simulink model "RBFNN"  (Simulink 10.0)
settings: Solver=VariableStepAuto  StartTime=0.0  StopTime=5  MaxStep=5e-4  RelTol=1e-3
undefined symbols (not defined in the file): ln
libraries: powerlib x14, powerlib_meascontrol x1
settings Model: Creator=guanc  LastModifiedBy=Administrator
settings SolverCC: AlgebraicLoopSolver=LineSearch
settings DataIOCC: SaveFormat=Dataset
settings OptimizationCC: LifeSpan=auto
settings DebuggingCC: UnderspecifiedInitializationDetection=Simplified  MergeDetectMultiDrivingBlocksExec=error  SFUnexpectedBacktrackingDiag=error  SFNoUnconditionalDefaultTransitionDiag=error  SFExecutionAtInitializationDiag=warning
settings HardwareCC: ProdBitPerPointer=64  ProdBitPerSizeT=64  ProdBitPerPtrDiffT=64  ProdLargestAtomicFloat=Float  ProdIntDivRoundTo=Zero  ProdEndianess=LittleEndian  ProdWordSize=64  ProdHWDeviceType=Intel->x86-64 (Windows64)
settings ModelReferenceCC: PropagateSignalLabelsOutOfModel=on
settings GRTTargetCC: TargetLangStandard=C99 (ISO)  CombineOutputUpdateFcns=on  GRTInterface=off
settings ConfigComp: CovMetricSettings=dwe  CovHtmlReporting=off  CovSaveCumulativeToWorkspaceVar=off  CovSaveSingleToWorkspaceVar=off
settings SimscapeCC: SimscapeNormalizeSystem=off

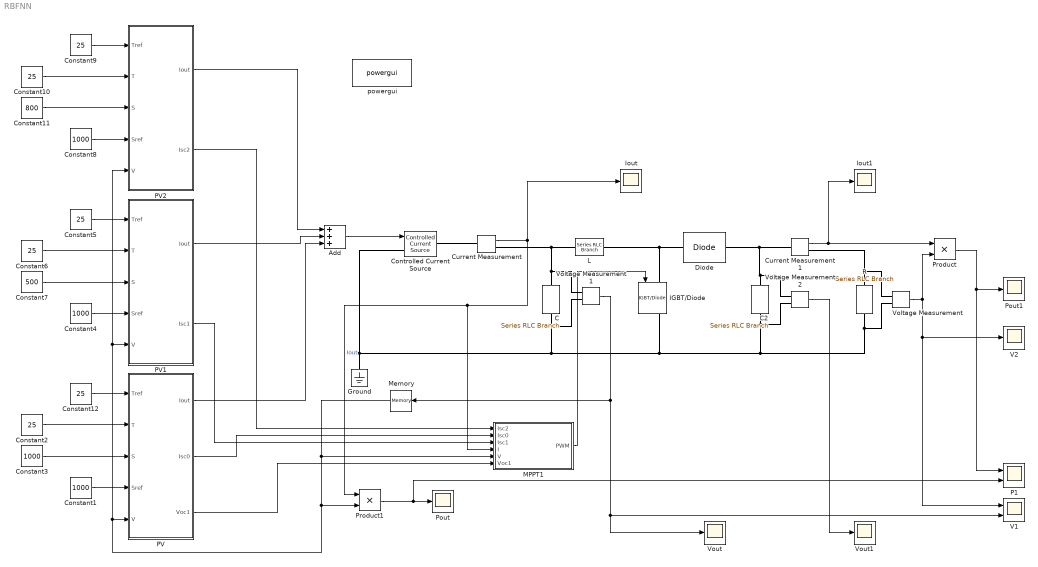
== system RBFNN ==
  Add : Sum  Inputs=+++
  C : powerlib/Elements/Series RLC Branch  LConnTagsString=__new0  RConnTagsString=__new0  BranchType=C  Resistance=1  Inductance=1e-3  SetiL0=off  InitialCurrent=0  Capacitance=47e-6  Setx0=off  InitialVoltage=1  Measurements=None
      settings: SourceProductName=Simscape Electrical
  C2 : powerlib/Elements/Series RLC Branch  LConnTagsString=__new0  RConnTagsString=__new0  BranchType=C  Resistance=1  Inductance=1e-3  SetiL0=off  InitialCurrent=0  Capacitance=470e-6  Setx0=off  InitialVoltage=1  Measurements=None
      settings: SourceProductName=Simscape Electrical
  Constant{1,3..4,8} (4 alike) : Constant  Value=1000
  Constant{2,5..6,9..10,12} (6 alike) : Constant  Value=25
  Constant11 : Constant  Value=800
  Constant7 : Constant  Value=500
  Controlled Current Source : powerlib/Electrical Sources/Controlled Current Source  Initialize=on  Source_Type=DC  Amplitude=0  Phase=0  Frequency=0  Measurements=None
      settings: SourceProductName=Simscape Electrical
  Current Measurement : powerlib/Measurements/Current Measurement  PhasorSimulation=off  OutputType=Complex  PSBequivalent=0
      settings: SourceProductName=Simscape Electrical
  Current Measurement1 : powerlib/Measurements/Current Measurement  PhasorSimulation=off  OutputType=Complex  PSBequivalent=0
      settings: SourceProductName=Simscape Electrical
  Diode : powerlib/Power Electronics/Diode  Ron=0.001  Lon=0  Vf=0.8  IC=0  UseSnubber=off  Rs=500  Cs=250e-9  Measurements=off
      settings: SourceProductName=Simscape Electrical
  Ground : powerlib/Elements/Ground  LConnTagsString=a
      settings: SourceProductName=Simscape Electrical
  IGBT/Diode : powerlib/Power Electronics/IGBT//Diode  Ron=1e-3  Rs=1e5  Cs=inf  Measurements=on
      settings: SourceProductName=Simscape Electrical
  Iout : Scope
  Iout1 : Scope
  L : powerlib/Elements/Series RLC Branch  LConnTagsString=__new0  RConnTagsString=__new0  BranchType=L  Resistance=1  Inductance=1e-3  SetiL0=off  InitialCurrent=0  Capacitance=1e-6  Setx0=off  InitialVoltage=0  Measurements=None
      settings: SourceProductName=Simscape Electrical
  MPPT1 : Subsystem
  Memory : Memory
  P1 : Scope  NumInputPorts=2
  PV : Subsystem  mask{a=0.0025, b=0.5, c=0.0028, Voc=21.8, Vm=17.7, Isc=3.64, Im=3.24}
      mask help: 根据电池铭牌参数设置
      mask TypeOptions a: a/Gain
      mask TypeOptions b: b/Gain
      mask TypeOptions c: c/Gain
      mask TypeOptions Voc: Voc/Value
      mask TypeOptions Vm: Vm/Value
      mask TypeOptions Isc: Isc/Value
      mask TypeOptions Im: Im/Value
  PV1 : Subsystem  mask{a=0.0025, b=0.5, c=0.0028, Voc=21.8, Vm=17.7, Isc=3.64, Im=3.24}
      mask help: 根据电池铭牌参数设置
      mask TypeOptions a: a/Gain
      mask TypeOptions b: b/Gain
      mask TypeOptions c: c/Gain
      mask TypeOptions Voc: Voc/Value
      mask TypeOptions Vm: Vm/Value
      mask TypeOptions Isc: Isc/Value
      mask TypeOptions Im: Im/Value
  PV2 : Subsystem  mask{a=0.0025, b=0.5, c=0.0028, Voc=21.8, Vm=17.7, Isc=3.64, Im=3.24}
      mask help: 根据电池铭牌参数设置
      mask TypeOptions a: a/Gain
      mask TypeOptions b: b/Gain
      mask TypeOptions c: c/Gain
      mask TypeOptions Voc: Voc/Value
      mask TypeOptions Vm: Vm/Value
      mask TypeOptions Isc: Isc/Value
      mask TypeOptions Im: Im/Value
  Pout : Scope
  Pout1 : Scope
  Product : Product
  Product1 : Product
  R : powerlib/Elements/Series RLC Branch  LConnTagsString=__new0  RConnTagsString=__new0  BranchType=R  Resistance=20  Inductance=1e-3  SetiL0=off  InitialCurrent=0  Capacitance=1e-6  Setx0=off  InitialVoltage=0  Measurements=None
      settings: SourceProductName=Simscape Electrical
  V1 : Scope  NumInputPorts=2
  V2 : Scope
  Voltage Measurement : powerlib/Measurements/Voltage Measurement  PhasorSimulation=off  OutputType=Complex  PSBequivalent=0
      settings: SourceProductName=Simscape Electrical
  Voltage Measurement1 : powerlib/Measurements/Voltage Measurement  PhasorSimulation=off  OutputType=Complex  PSBequivalent=0
      settings: SourceProductName=Simscape Electrical
  Voltage Measurement2 : powerlib/Measurements/Voltage Measurement  PhasorSimulation=off  OutputType=Complex  PSBequivalent=0
      settings: SourceProductName=Simscape Electrical
  Vout : Scope
  Vout1 : Scope
  powergui : powerlib/powergui  Priority=1  SimulationMode=Discrete  SampleTime=5e-6  frequency=60  Iterations=50  frequencyindice=0  Pbase=100e6  ErrMax=1e-4  UnitsV=kV  UnitsW=MW  buscounter=0  FunctionMessages=off  echomessages=off  EnableUseOfTLC=off  CurrentSourceSwitches=on  DisableSnubberDevices=off  DisableRonSwitches=off  DisableVfSwitches=off  DisplayEquations=off  AutomaticDiscreteSolvers=off  SolverType=Tustin/Backward Euler (TBE)  Interpol=off  ExternalGateDelay=off  methode=off  Ts=0  x0status=blocks  SPID=off  SwTol=0  HookPort=off  NonlinearTolerance=1e-4  nMaxIteration=100  ContinueOnMaxIteration=off  RestoreLinks=warning  ResistiveCurrentMeasurement=off  Frange=[0:2:500]  Ylog=off  Xlog=on  ShowGrid=off  save=off  variable=ZData  structure=0  ZoomFFT=off  StartTime=0.0  cycles=1  DisplayStyle=1  fundamental=60  FreqAxis=off  MaxFrequency=1000  frequencyindicesteady=1  RmsSteady=1  display=off
      settings: SourceProductName=Simscape Electrical
  wires:
  Current Measurement1/1 -> Iout1/1, Product/1
  Voltage Measurement/1 -> V2/1, V1/1, Product/2
  Product/1 -> P1/1, Pout1/1
  Current Measurement/1 -> MPPT1/4(I), Product1/1, Iout/1  "Iout"
  MPPT1/1(PWM) -> IGBT/Diode/1
  Product1/1 -> P1/2, Pout/1
  Voltage Measurement2/1 -> Vout1/1
  Voltage Measurement1/1 -> Memory/1, Vout/1, V1/2
  Constant3/1 -> PV/3(S)
  Constant12/1 -> PV/1(Tref)
  PV/1(Iout) -> Add/3
  Constant2/1 -> PV/2(T)
  Constant1/1 -> PV/4(Sref)
  Constant4/1 -> PV1/4(Sref)
  Constant6/1 -> PV1/2(T)
  Constant5/1 -> PV1/1(Tref)
  Constant7/1 -> PV1/3(S)
  Constant8/1 -> PV2/4(Sref)
  Constant10/1 -> PV2/2(T)
  Constant9/1 -> PV2/1(Tref)
  Constant11/1 -> PV2/3(S)
  Add/1 -> Controlled Current Source/1
  PV2/1(Iout) -> Add/1
  PV1/1(Iout) -> Add/2
  Memory/1 -> PV/5(V), PV1/5(V), PV2/5(V), Product1/2, MPPT1/5(V)
  PV/2(Isc0) -> MPPT1/2(Isc0)
  PV2/2(Isc2) -> MPPT1/1(Isc2)
  PV1/2(Isc1) -> MPPT1/3(Isc1)
  PV/3(Voc1) -> MPPT1/6(Voc1)
  connections:
  C/RConn1 -- Voltage Measurement1/LConn2 -- Controlled Current Source/LConn1 -- Ground/LConn1 -- Voltage Measurement2/LConn2 -- C2/RConn1 -- Voltage Measurement/LConn2 -- R/RConn1 -- IGBT/Diode/RConn1
  Voltage Measurement1/LConn1 -- C/LConn1 -- Current Measurement/RConn1 -- L/LConn1
  IGBT/Diode/LConn1 -- L/RConn1 -- Diode/LConn1
  Voltage Measurement2/LConn1 -- Diode/RConn1 -- Current Measurement1/LConn1 -- C2/LConn1
  R/LConn1 -- Voltage Measurement/LConn1 -- Current Measurement1/RConn1
  Controlled Current Source/RConn1 -- Current Measurement/LConn1

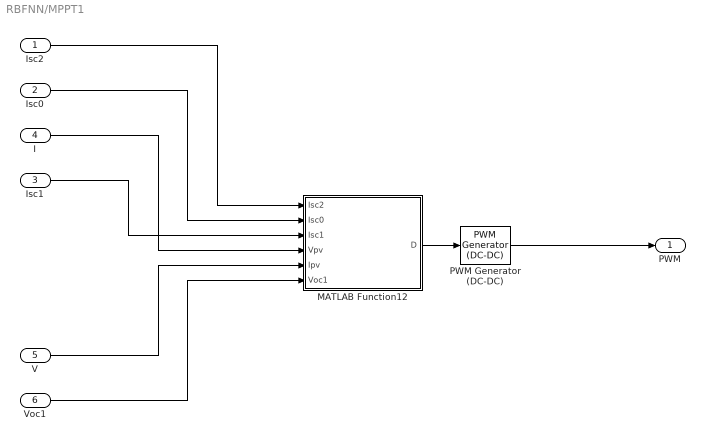
== system RBFNN/MPPT1 ==
  Isc2 : Inport
  Isc0 : Inport  Port=2
  Isc1 : Inport  Port=3
  I : Inport  Port=4
  V : Inport  Port=5
  Voc1 : Inport  Port=6
  MATLAB Function12 : MATLAB Function  TreatAsAtomicUnit=on
  PWM Generator (DC-DC) : powerlib_meascontrol/Pulse & Signal Generators/PWM Generator (DC-DC)  Fsw=1e4  Ts=0
      settings: SourceProductName=Simscape Electrical
  PWM : Outport
  wires:
  I/1 -> MATLAB Function12/4(Vpv)
  V/1 -> MATLAB Function12/5(Ipv)
  PWM Generator (DC-DC)/1 -> PWM/1
  MATLAB Function12/1(D) -> PWM Generator (DC-DC)/1
  Isc2/1 -> MATLAB Function12/1(Isc2)
  Isc0/1 -> MATLAB Function12/2(Isc0)
  Isc1/1 -> MATLAB Function12/3(Isc1)
  Voc1/1 -> MATLAB Function12/6(Voc1)

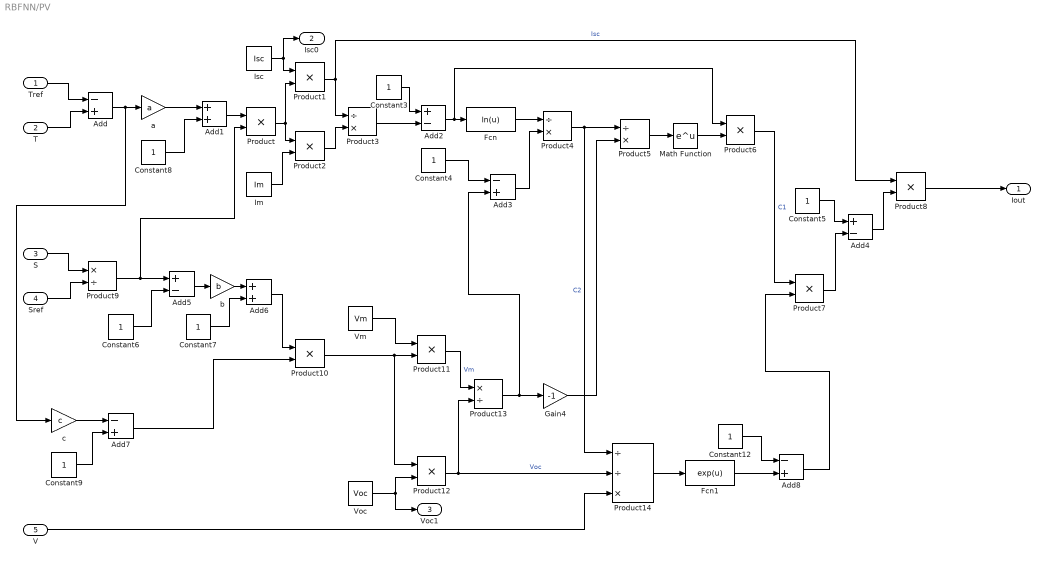
== system RBFNN/PV ==
  Tref : Inport
  T : Inport  Port=2
  S : Inport  Port=3
  Sref : Inport  Port=4
  V : Inport  Port=5
  Add{,3,7..8} (4 alike) : Sum  Inputs=-+
  Add1 : Sum
  Add2 : Sum  Inputs=+-
  Add4 : Sum  Inputs=+-
  Add5 : Sum  Inputs=+-
  Add6 : Sum
  Constant{3..9,12} (8 alike) : Constant
  Fcn : Fcn  Expr=ln(u)
  Fcn1 : Fcn  Expr=exp(u)
  Gain4 : Gain  Gain=-1  OutDataTypeStr=Inherit: Same as input  ParamDataTypeStr=Inherit: Same as input
  Im : Constant  Value=Im
  Isc : Constant  Value=Isc
  Math Function : Math  SaturateOnIntegerOverflow=on
  Product{,1..2,6..8,10..12} (9 alike) : Product
  Product13 : Product  Inputs=*/
  Product14 : Product  Inputs=//*
  Product3 : Product  Inputs=/*
  Product4 : Product  Inputs=/*
  Product5 : Product  Inputs=/*
  Product9 : Product  Inputs=*/
  Vm : Constant  Value=Vm
  Voc : Constant  Value=Voc
  a : Gain  Gain=a  OutDataTypeStr=Inherit: Same as input  ParamDataTypeStr=Inherit: Same as input
  b : Gain  Gain=b  OutDataTypeStr=Inherit: Same as input  ParamDataTypeStr=Inherit: Same as input
  c : Gain  Gain=c  OutDataTypeStr=Inherit: Same as input  ParamDataTypeStr=Inherit: Same as input
  Iout : Outport
  Isc0 : Outport  Port=2
  Voc1 : Outport  Port=3
  wires:
  Math Function/1 -> Product6/2
  Product1/1 -> Product8/1, Product3/1  "Isc"
  Tref/1 -> Add/1
  Sref/1 -> Product9/2
  Constant9/1 -> Add7/2
  c/1 -> Add7/1
  Add6/1 -> Product10/1
  Product10/1 -> Product11/2, Product12/1
  Constant6/1 -> Add5/2
  Voc/1 -> Voc1/1, Product12/2
  T/1 -> Add/2
  b/1 -> Add6/1
  Product13/1 -> Add3/2, Gain4/1
  Product8/1 -> Iout/1
  Product9/1 -> Product/2, Add5/1
  Product11/1 -> Product13/1  "Vm"
  Add4/1 -> Product8/2
  Add3/1 -> Product4/2
  Product2/1 -> Product3/2
  Product/1 -> Product2/1, Product1/2
  Product4/1 -> Product14/1, Product5/1  "C2"
  Constant3/1 -> Add2/1
  Product5/1 -> Math Function/1
  Constant7/1 -> Add6/2
  Add5/1 -> b/1
  Add8/1 -> Product7/2
  Add1/1 -> Product/1
  Constant8/1 -> Add1/2
  Constant4/1 -> Add3/1
  Fcn/1 -> Product4/1
  Product6/1 -> Product7/1  "C1"
  S/1 -> Product9/1
  Vm/1 -> Product11/1
  Constant5/1 -> Add4/1
  Add2/1 -> Product6/1, Fcn/1
  Gain4/1 -> Product5/2
  Product3/1 -> Add2/2
  a/1 -> Add1/1
  Product7/1 -> Add4/2
  Isc/1 -> Product1/1, Isc0/1
  Constant12/1 -> Add8/1
  Im/1 -> Product2/2
  Product12/1 -> Product14/2, Product13/2  "Voc"
  Add7/1 -> Product10/2
  Add/1 -> c/1, a/1
  V/1 -> Product14/3
  Product14/1 -> Fcn1/1
  Fcn1/1 -> Add8/2

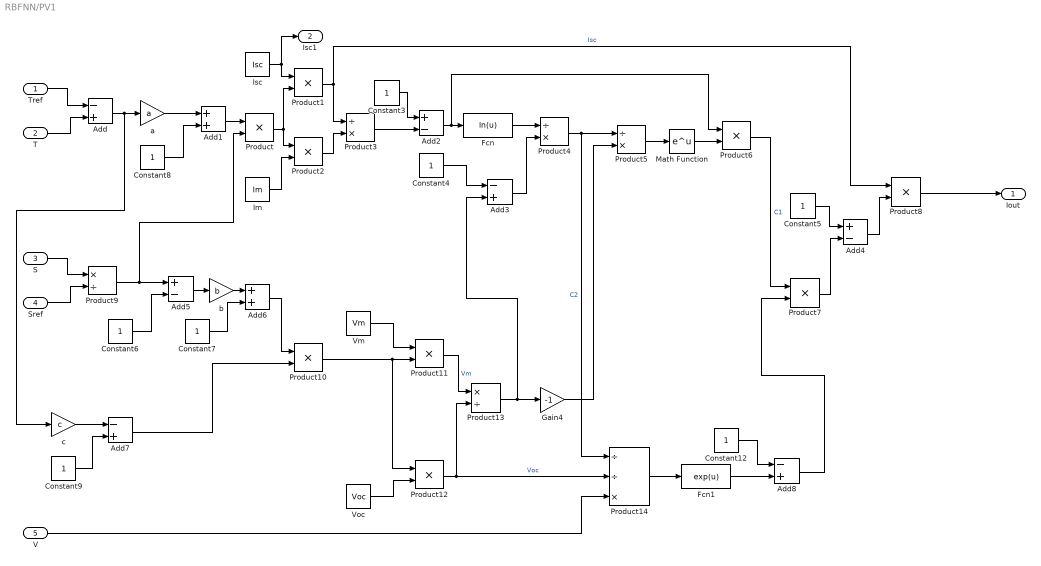
== system RBFNN/PV1 ==
  Tref : Inport
  T : Inport  Port=2
  S : Inport  Port=3
  Sref : Inport  Port=4
  V : Inport  Port=5
  Add{,3,7..8} (4 alike) : Sum  Inputs=-+
  Add1 : Sum
  Add2 : Sum  Inputs=+-
  Add4 : Sum  Inputs=+-
  Add5 : Sum  Inputs=+-
  Add6 : Sum
  Constant{3..9,12} (8 alike) : Constant
  Fcn : Fcn  Expr=ln(u)
  Fcn1 : Fcn  Expr=exp(u)
  Gain4 : Gain  Gain=-1  OutDataTypeStr=Inherit: Same as input  ParamDataTypeStr=Inherit: Same as input
  Im : Constant  Value=Im
  Isc : Constant  Value=Isc
  Math Function : Math  SaturateOnIntegerOverflow=on
  Product{,1..2,6..8,10..12} (9 alike) : Product
  Product13 : Product  Inputs=*/
  Product14 : Product  Inputs=//*
  Product3 : Product  Inputs=/*
  Product4 : Product  Inputs=/*
  Product5 : Product  Inputs=/*
  Product9 : Product  Inputs=*/
  Vm : Constant  Value=Vm
  Voc : Constant  Value=Voc
  a : Gain  Gain=a  OutDataTypeStr=Inherit: Same as input  ParamDataTypeStr=Inherit: Same as input
  b : Gain  Gain=b  OutDataTypeStr=Inherit: Same as input  ParamDataTypeStr=Inherit: Same as input
  c : Gain  Gain=c  OutDataTypeStr=Inherit: Same as input  ParamDataTypeStr=Inherit: Same as input
  Iout : Outport
  Isc1 : Outport  Port=2
  wires:
  Math Function/1 -> Product6/2
  Product1/1 -> Product8/1, Product3/1  "Isc"
  Tref/1 -> Add/1
  Sref/1 -> Product9/2
  Constant9/1 -> Add7/2
  c/1 -> Add7/1
  Add6/1 -> Product10/1
  Product10/1 -> Product11/2, Product12/1
  Constant6/1 -> Add5/2
  Voc/1 -> Product12/2
  T/1 -> Add/2
  b/1 -> Add6/1
  Product13/1 -> Add3/2, Gain4/1
  Product8/1 -> Iout/1
  Product9/1 -> Product/2, Add5/1
  Product11/1 -> Product13/1  "Vm"
  Add4/1 -> Product8/2
  Add3/1 -> Product4/2
  Product2/1 -> Product3/2
  Product/1 -> Product2/1, Product1/2
  Product4/1 -> Product14/1, Product5/1  "C2"
  Constant3/1 -> Add2/1
  Product5/1 -> Math Function/1
  Constant7/1 -> Add6/2
  Add5/1 -> b/1
  Add8/1 -> Product7/2
  Add1/1 -> Product/1
  Constant8/1 -> Add1/2
  Constant4/1 -> Add3/1
  Fcn/1 -> Product4/1
  Product6/1 -> Product7/1  "C1"
  S/1 -> Product9/1
  Vm/1 -> Product11/1
  Constant5/1 -> Add4/1
  Add2/1 -> Product6/1, Fcn/1
  Gain4/1 -> Product5/2
  Product3/1 -> Add2/2
  a/1 -> Add1/1
  Product7/1 -> Add4/2
  Isc/1 -> Product1/1, Isc1/1
  Constant12/1 -> Add8/1
  Im/1 -> Product2/2
  Product12/1 -> Product14/2, Product13/2  "Voc"
  Add7/1 -> Product10/2
  Add/1 -> c/1, a/1
  V/1 -> Product14/3
  Product14/1 -> Fcn1/1
  Fcn1/1 -> Add8/2

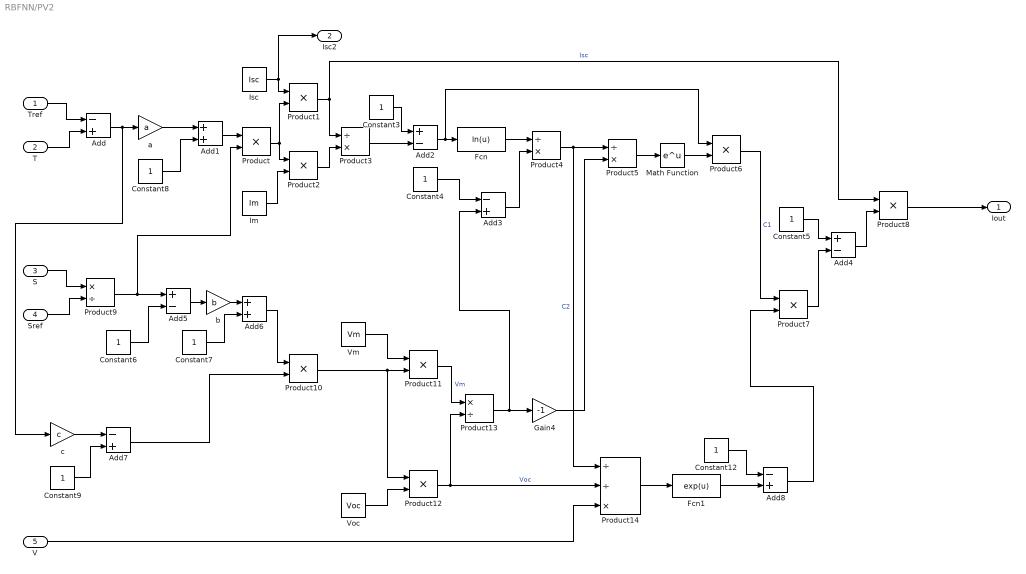
== system RBFNN/PV2 ==
  Tref : Inport
  T : Inport  Port=2
  S : Inport  Port=3
  Sref : Inport  Port=4
  V : Inport  Port=5
  Add{,3,7..8} (4 alike) : Sum  Inputs=-+
  Add1 : Sum
  Add2 : Sum  Inputs=+-
  Add4 : Sum  Inputs=+-
  Add5 : Sum  Inputs=+-
  Add6 : Sum
  Constant{3..9,12} (8 alike) : Constant
  Fcn : Fcn  Expr=ln(u)
  Fcn1 : Fcn  Expr=exp(u)
  Gain4 : Gain  Gain=-1  OutDataTypeStr=Inherit: Same as input  ParamDataTypeStr=Inherit: Same as input
  Im : Constant  Value=Im
  Isc : Constant  Value=Isc
  Math Function : Math  SaturateOnIntegerOverflow=on
  Product{,1..2,6..8,10..12} (9 alike) : Product
  Product13 : Product  Inputs=*/
  Product14 : Product  Inputs=//*
  Product3 : Product  Inputs=/*
  Product4 : Product  Inputs=/*
  Product5 : Product  Inputs=/*
  Product9 : Product  Inputs=*/
  Vm : Constant  Value=Vm
  Voc : Constant  Value=Voc
  a : Gain  Gain=a  OutDataTypeStr=Inherit: Same as input  ParamDataTypeStr=Inherit: Same as input
  b : Gain  Gain=b  OutDataTypeStr=Inherit: Same as input  ParamDataTypeStr=Inherit: Same as input
  c : Gain  Gain=c  OutDataTypeStr=Inherit: Same as input  ParamDataTypeStr=Inherit: Same as input
  Iout : Outport
  Isc2 : Outport  Port=2
  wires:
  Math Function/1 -> Product6/2
  Product1/1 -> Product8/1, Product3/1  "Isc"
  Tref/1 -> Add/1
  Sref/1 -> Product9/2
  Constant9/1 -> Add7/2
  c/1 -> Add7/1
  Add6/1 -> Product10/1
  Product10/1 -> Product11/2, Product12/1
  Constant6/1 -> Add5/2
  Voc/1 -> Product12/2
  T/1 -> Add/2
  b/1 -> Add6/1
  Product13/1 -> Add3/2, Gain4/1
  Product8/1 -> Iout/1
  Product9/1 -> Product/2, Add5/1
  Product11/1 -> Product13/1  "Vm"
  Add4/1 -> Product8/2
  Add3/1 -> Product4/2
  Product2/1 -> Product3/2
  Product/1 -> Product2/1, Product1/2
  Product4/1 -> Product14/1, Product5/1  "C2"
  Constant3/1 -> Add2/1
  Product5/1 -> Math Function/1
  Constant7/1 -> Add6/2
  Add5/1 -> b/1
  Add8/1 -> Product7/2
  Add1/1 -> Product/1
  Constant8/1 -> Add1/2
  Constant4/1 -> Add3/1
  Fcn/1 -> Product4/1
  Product6/1 -> Product7/1  "C1"
  S/1 -> Product9/1
  Vm/1 -> Product11/1
  Constant5/1 -> Add4/1
  Add2/1 -> Product6/1, Fcn/1
  Gain4/1 -> Product5/2
  Product3/1 -> Add2/2
  a/1 -> Add1/1
  Product7/1 -> Add4/2
  Isc/1 -> Product1/1, Isc2/1
  Constant12/1 -> Add8/1
  Im/1 -> Product2/2
  Product12/1 -> Product14/2, Product13/2  "Voc"
  Add7/1 -> Product10/2
  Add/1 -> c/1, a/1
  V/1 -> Product14/3
  Product14/1 -> Fcn1/1
  Fcn1/1 -> Add8/2

== matlab function MPPT1/MATLAB Function12 ==
  data: Isc2 input double; Isc0 input double; Isc1 input double; Vpv input double; D output double; Ipv input double; Voc1 input double
function D = NNIDA_code(Isc2, Isc0, Isc1, Vpv,Ipv, Voc1)

persistent Food_fitness Enemy_fitness Food_pos Enemy_pos X DeltaX Neighbours_DeltaX Neighbours_X Fitness;
%display('IDA is optimizing your problem');

SearchAgents_no = 10;
Max_iteration = 100;
lb = 0.1;
ub = 0.9;
dim = 1;
test_out = inf;

strength=1;
if nargin<2
    strength=1;
end 
u=[Isc2;Isc0;Isc1;Voc1];
d=u.';
output=(u.'-mean(u.'))*strength./(max(u.')-min(u.'));
out=output.';
size_te=size(out,4);  
in_num=4;          
[hid_num,w,b,c]=load ('net_RBF_UserDefined.mat')     
h=zeros(hid_num,1);

for i=1:size_te
    for k=1:hid_num
        l=1:4
        h(k)=exp(-norm(out(l,i)-c(k,1))^2/(2*b(k)^2));
    end
    test_out(i)=w*h;
end

%The initial radius of gragonflies' neighbourhoods
r=(ub-lb)/10;
Delta_max=(ub-lb)/10;

if(isempty(Food_fitness))
    Food_fitness = zeros(dim,1);
end

if(isempty(Enemy_fitness))
    Enemy_fitness = zeros(dim,1);
end

if(isempty(Food_pos))
    Food_pos = zeros(SearchAgents_no,1);
end

if(isempty(Enemy_pos))
    Enemy_pos = zeros(SearchAgents_no,1);
end

if(isempty(Fitness))
    Fitness = zeros(SearchAgents_no,1);
end

X=initialization(SearchAgents_no,dim,ub,lb);

DeltaX=initialization(SearchAgents_no,dim,ub,lb);

Neighbours_DeltaX = zeros(SearchAgents_no,1);
Neighbours_X = zeros(SearchAgents_no,1);

for iter=1:Max_iteration
    
    r=(ub-lb)/4+((ub-lb)*(iter/Max_iteration)*2);
    
    w=0.9-iter*((0.9-0.4)/Max_iteration);
       
    my_c=0.1-iter*((0.1-0)/(Max_iteration/2));
    if my_c<0
        my_c=0;
    end
    s=2*rand*my_c; 
    a=2*rand*my_c; 
    c=2*rand*my_c; 
    f=2*rand;      
    e=my_c;       
    
    for i=1:SearchAgents_no 
        Fitness(i,1)=-(test_out*Ipv);
        if Fitness(i,1)<Food_fitness
            Food_fitness=Fitness(i,1);
            Food_pos=X(i,:);
        end
        
        if Fitness(i,1)>Enemy_fitness
            if all(X(i,:)<ub') && all( X(i,:)>lb')
                Enemy_fitness=Fitness(i,1);
                Enemy_pos=X(i,:);
            end
        end
    end
    
    for i=1:SearchAgents_no
        index=0;
        neighbours_no=0;
        
         for j=1:SearchAgents_no
            Dist2Enemy=distance(X(i,:),X(j,:));
            if (all(Dist2Enemy<=r) && all(Dist2Enemy~=0))
                index=index+1;
                neighbours_no=neighbours_no+1;
                Neighbours_DeltaX(index,:)=DeltaX(j,:);
                Neighbours_X(index,:)=X(j,:);
            end
        end
        
        S=zeros(dim,1);
        if neighbours_no>1
            for k=1:neighbours_no
                S=S+(Neighbours_X(k,:)-X(i,:));
            end
            S=-S;
        else
            S=zeros(dim,1);
        end
        
        if neighbours_no>1
            A=(sum(Neighbours_DeltaX')')/neighbours_no;
        else
            A=DeltaX(i,:);
        end
        
        if neighbours_no>1
            C_temp=(sum(Neighbours_X')')/neighbours_no;
        else
            C_temp=X(i,:);
        end
        
        C=C_temp-X(i,:);
        
        Dist2Food=distance(X(i,:),Food_pos(:,1));
        if all(Dist2Food<=r)
            F=Food_pos-X(i,:);
        else
            F=0;
        end
        
        Dist2Enemy=distance(X(i,:),Enemy_pos(:,1));
        if all(Dist2Enemy<=r)
            Enemy=Enemy_pos+X(i,:);
        else
            Enemy=zeros(dim,1);
        end
        
        for tt=1:dim
            if X(i,tt)>ub(tt)
                X(i,tt)=lb(tt);
                DeltaX(i,tt)=rand;
            end
            if X(i,tt)<lb(tt)
                X(i,tt)=ub(tt);
                DeltaX(i,tt)=rand;
            end
        end
        
        if any(Dist2Food>r)
            if neighbours_no>1
                for j=1:dim
                    DeltaX(i,j)=w*DeltaX(i,j)+rand*A(j,1)+rand*C(j,1)+rand*S(j,1);
                    if DeltaX(i,j)>Delta_max(j)
                        DeltaX(i,j)=Delta_max(j);
                    end
                    if DeltaX(i,j)<-Delta_max(j)
                        DeltaX(i,j)=-Delta_max(j);
                    end
                    X(i,j)=X(i,j)+DeltaX(i,j);
                end
            else
 
                X(i,:)=X(i,:)+Levy(dim)'.*X(i,:);
                DeltaX(i,:)=0;
            end
        else
            for j=1:dim

                DeltaX(i,j)=(a*A(j,1)+c*C(j,1)+s*S(j,1)+f*F(j,1)+e*Enemy(j,1)) + w*DeltaX(i,j);
                if DeltaX(i,j)>Delta_max(j)
                    DeltaX(i,j)=Delta_max(j);
                end
                if DeltaX(i,j)<-Delta_max(j)
                    DeltaX(i,j)=-Delta_max(j);
                end
                X(i,j)=X(i,j)+DeltaX(i,j);
            end 
        end
        
        if(Food_pos > ub)
            Food_pos=ub;
        end
        if(Food_pos < lb)
            Food_pos=lb;
        end
    end
    %Best_score=Food_fitness;     
    [~,idx] = min(Food_fitness);
    D=Food_pos(1,:);
end
end

function Positions=initialization(SearchAgents_no,dim,ub,lb)
Positions=zeros(SearchAgents_no,1);
Boundary_no= size(ub,2); 

if Boundary_no==1
    ub_new=ones(1,dim)*ub;
    lb_new=ones(1,dim)*lb;
else
     ub_new=ub;
     lb_new=lb;   
end
    for i=1:dim
        ub_i=ub_new(i);
        lb_i=lb_new(i);
        Positions=rand(SearchAgents_no,1).*(ub_i-lb_i)+lb_i;
    end
Positions=Positions;
end


function o = distance(a,b)
o = zeros(1);
for i=1:1
    o(i,1)=sqrt((a(i)-b(i))^2);
end
end

function o=Levy(d)
beta=3/2;

sigma=(gamma(1+beta)*sin(pi*beta/2)/(gamma((1+beta)/2)*beta*2^((beta-1)/2)))^(1/beta);
u=randn(1,d)*sigma;
v=randn(1,d);
step=u./abs(v).^(1/beta);

o=0.01*step;
end
